simulink model "T2t"  (Simulink 8.4)
settings: Solver=ode45  StartTime=0.0  StopTime=10.0  RelTol=1e-3
undefined symbols (not defined in the file): T2t_facKThrValveReqCorr, T2t_facThrValveReqCorrEnable, T2t_facWastegateReqCorrEnable, T2t_KWastegateReqCorr, T2t_pManiReqMan, T2t_pManiReqMin, T2t_pManiReqOverride, T2t_pManiRes, T2t_ThrPosStart, T2t_ThrValve2WasteGateThreshold, T2t_ThrValveReqCorrMax, T2t_ThrValveReqCorrMin, T2t_tiTnThrValveReqCorr, T2t_tiTnWastegateReqCorr, T2t_tiTvThrValveReqCorr, T2t_tiTvWastegateReqCorr
libraries: simulink x5
settings Model: Creator=YAL9FE  LastModifiedBy=ric9fe
settings DebuggingCC: FcnCallInpInsideContextMsg=EnableAllAsWarning

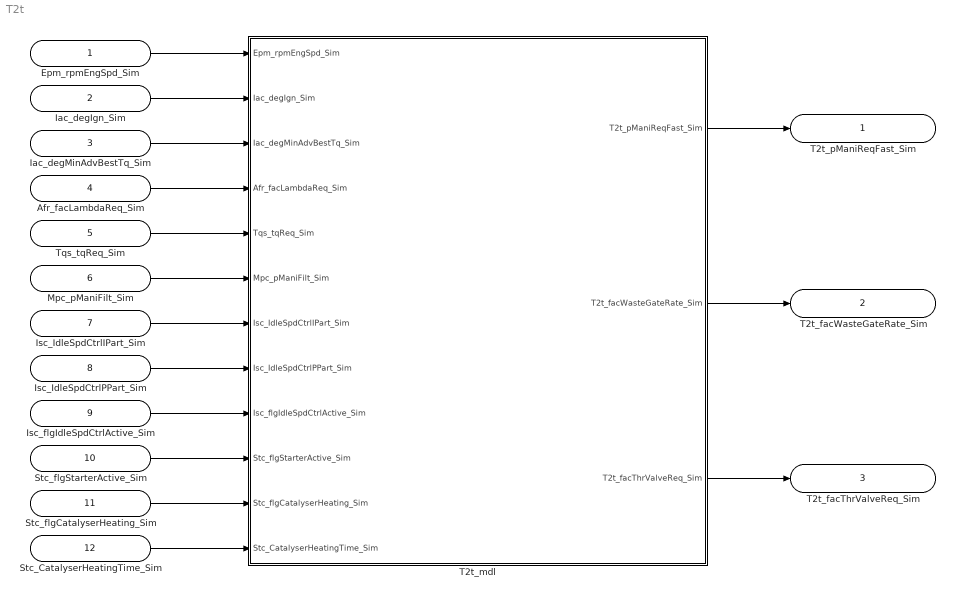
== system T2t ==
  Epm_rpmEngSpd_Sim : Inport
  Iac_degIgn_Sim : Inport  Port=2
  Iac_degMinAdvBestTq_Sim : Inport  Port=3
  Afr_facLambdaReq_Sim : Inport  Port=4
  Tqs_tqReq_Sim : Inport  Port=5
  Mpc_pManiFilt_Sim : Inport  Port=6
  Isc_IdleSpdCtrlIPart_Sim : Inport  Port=7
  Isc_IdleSpdCtrlPPart_Sim : Inport  Port=8
  Isc_flgIdleSpdCtrlActive_Sim : Inport  Port=9
  Stc_flgStarterActive_Sim : Inport  Port=10
  Stc_flgCatalyserHeating_Sim : Inport  Port=11
  Stc_CatalyserHeatingTime_Sim : Inport  Port=12
  T2t_mdl : Subsystem  mask(Functions){}
      mask help: Torque2Throttle
      mask Display:
      | image(imread('Torque2Throttle.jpg'))
      | port_label('input',1,'Epm_rpmEngSpd_Sim')
      | port_label('input',2,'Iac_degIgn_Sim')
      | port_label('input',3,'Iac_degMinAdvBestTq_Sim')
      | port_label('input',4,'Afr_facLambdaReq_Sim')
      | port_label('input',5,'Tqs_tqReq_Sim')
      | port_label('input',6,'Mpc_pManiFilt_Sim')
      | port_label('input',7,'Isc_IdleSpdCtrlIPart_Sim')
      | port_label('input',8,'Isc_IdleSpdCtrlPPart_Sim')
      | port_label('input',9,'Isc_flgIdleSpdCtrlActive_Sim')
      | port_label('input',10,'Stc_flgStarterActive_Sim')
      | port_label('input',11,'Stc_flgCatalyserHeating_Sim')
      | port_label('input',12,'Stc_CatalyserHeatingTime_Sim')
      | port_label('output',1,'T2t_pManiReqFast_Sim')
      | port_label('output',2,'T2t_facWasteGateRate_Sim')
      | port_label('output',3,'T2t_facThrValveReq_Sim')
  T2t_pManiReqFast_Sim : Outport
  T2t_facWasteGateRate_Sim : Outport  Port=2
  T2t_facThrValveReq_Sim : Outport  Port=3
  wires:
  Epm_rpmEngSpd_Sim/1 -> T2t_mdl/1(Epm_rpmEngSpd_Sim)
  Iac_degIgn_Sim/1 -> T2t_mdl/2(Iac_degIgn_Sim)
  Iac_degMinAdvBestTq_Sim/1 -> T2t_mdl/3(Iac_degMinAdvBestTq_Sim)
  Afr_facLambdaReq_Sim/1 -> T2t_mdl/4(Afr_facLambdaReq_Sim)
  Tqs_tqReq_Sim/1 -> T2t_mdl/5(Tqs_tqReq_Sim)
  Mpc_pManiFilt_Sim/1 -> T2t_mdl/6(Mpc_pManiFilt_Sim)
  Isc_IdleSpdCtrlIPart_Sim/1 -> T2t_mdl/7(Isc_IdleSpdCtrlIPart_Sim)
  Isc_IdleSpdCtrlPPart_Sim/1 -> T2t_mdl/8(Isc_IdleSpdCtrlPPart_Sim)
  Isc_flgIdleSpdCtrlActive_Sim/1 -> T2t_mdl/9(Isc_flgIdleSpdCtrlActive_Sim)
  Stc_flgStarterActive_Sim/1 -> T2t_mdl/10(Stc_flgStarterActive_Sim)
  Stc_flgCatalyserHeating_Sim/1 -> T2t_mdl/11(Stc_flgCatalyserHeating_Sim)
  Stc_CatalyserHeatingTime_Sim/1 -> T2t_mdl/12(Stc_CatalyserHeatingTime_Sim)
  T2t_mdl/1(T2t_pManiReqFast_Sim) -> T2t_pManiReqFast_Sim/1
  T2t_mdl/2(T2t_facWasteGateRate_Sim) -> T2t_facWasteGateRate_Sim/1
  T2t_mdl/3(T2t_facThrValveReq_Sim) -> T2t_facThrValveReq_Sim/1

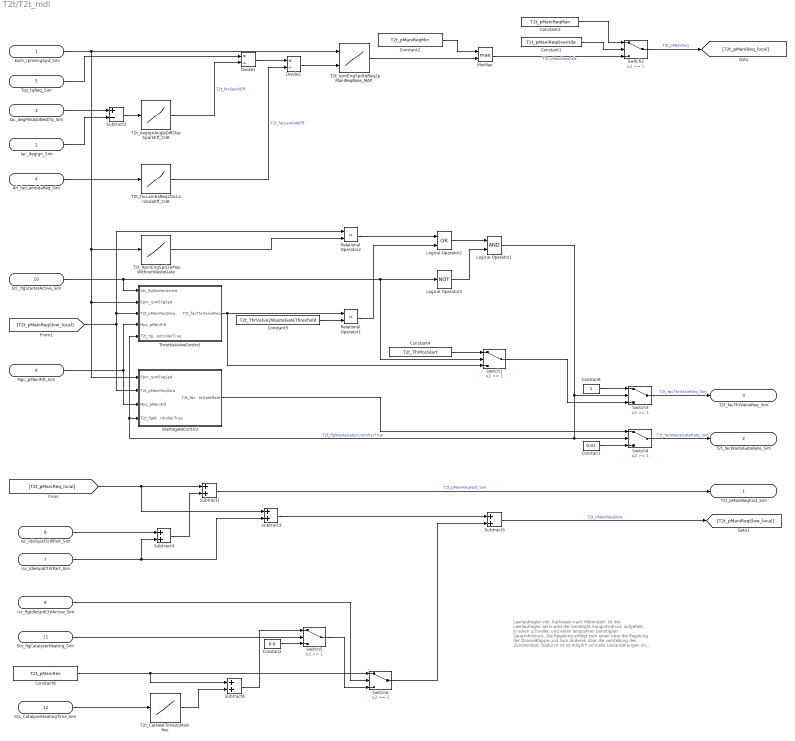
== system T2t/T2t_mdl ==
  note: Leerlaufregler inkl. Katheizen nach Motorstart:
      | Ist der Leerlaufregler aktiv wird der benötigte
      | Saugrohrdruck aufgeteilt, in einen schnellen
      | und einen langsamen benötigten Saugrohrdruck.
      | Die Regelung erfolgt zum einen über die
      | Regelung der Drosselklappe und zum anderen
      | über die verstellung des Zündwinkels.
      | Dadurch ist es möglich schnelle
      | Laständerungen im Leerlauf
      | durch Zündwinkeländerung auszuregeln.
      | Damit durch Zündwinkeländerung eine höhere
      | Momentenabgabe möglich ist, wird der
      | Saugrohrdruck erhöht um eine spätere
      | Zündung zu erhalten. Der
      | Zündwinkelwirkungsgrad wird niedriger.
      | Dadurch ist eine Momentenreserve vorhanden.
      |
      |
      | Der langsame Saugrohrdruck wird durch den
      | I-Anteil des Leerlaufreglers korrigiert.
      | Außerdem wird die Saugrohrdruckreserve addiert.
      | Der schnelle Saugrohrdruck wird durch den
      | P- und den I-Anteil des Leerlaufreglers korrigiert.
  Epm_rpmEngSpd_Sim : Inport
  Iac_degIgn_Sim : Inport  Port=2
  Iac_degMinAdvBestTq_Sim : Inport  Port=3
  Afr_facLambdaReq_Sim : Inport  Port=4
  Tqs_tqReq_Sim : Inport  Port=5
  Mpc_pManiFilt_Sim : Inport  Port=6
  Isc_IdleSpdCtrlIPart_Sim : Inport  Port=7
  Isc_IdleSpdCtrlPPart_Sim : Inport  Port=8
  Isc_flgIdleSpdCtrlActive_Sim : Inport  Port=9
  Stc_flgStarterActive_Sim : Inport  Port=10
  Stc_flgCatalyserHeating_Sim : Inport  Port=11
  Stc_CatalyserHeatingTime_Sim : Inport  Port=12
  Constan1 : Constant  Value=0.01  OutDataTypeStr=single
  Constan2 : Constant  Value=0.0  OutDataTypeStr=single
  Constan8 : Constant  OutDataTypeStr=single
  Constant1 : Constant  Value=T2t_pManiReqOverride
  Constant2 : Constant  Value=T2t_pManiReqMin
  Constant3 : Constant  Value=T2t_pManiReqMan
  Constant4 : Constant  Value=T2t_ThrPosStart
  Constant5 : Constant  Value=T2t_ThrValve2WasteGateThreshold
  Constant6 : Constant  Value=T2t_pManiRes
  Divide1 : Product  Inputs=*/  OutDataTypeStr=Inherit: Same as first input
  Divide2 : Product  Inputs=*/  OutDataTypeStr=Inherit: Same as first input
  Logical Operator1 : Logic  AllPortsSameDT=off  OutDataTypeStr=boolean
  Logical Operator2 : Logic  Operator=OR  AllPortsSameDT=off  OutDataTypeStr=boolean
  Logical Operator3 : Logic  Operator=NOT  AllPortsSameDT=off  OutDataTypeStr=boolean
  MinMax : MinMax  Function=max  Inputs=2
  Relational Operator1 : RelationalOperator  Operator=>  OutDataTypeStr=boolean
  Relational Operator2 : RelationalOperator  Operator=>  OutDataTypeStr=boolean
  Subtract{1,3..6} (5 alike) : Sum  OutDataTypeStr=Inherit: Same as first input
  Subtract2 : Sum  Inputs=+-  OutDataTypeStr=Inherit: Same as first input
  Switch{1..6} (6 alike) : Switch  Threshold=1
  T2t_CatHeatTime2pManiRes : Lookup_n-D  NumberOfTableDimensions=1  BreakpointsForDimension1=[1:3]  Table=[2 6 9]  ExtrapMethod=Clip  InputSameDT=on
  T2t_RpmEngSpd2pMaxWithoutWasteGate : Lookup_n-D  NumberOfTableDimensions=1  BreakpointsForDimension1=[1:3]  Table=[6 4 3]  ExtrapMethod=Clip  InputSameDT=on
  T2t_degIgnAngleDiff2facSparkEff_CUR : Lookup_n-D  NumberOfTableDimensions=1  BreakpointsForDimension1=[1:3]  Table=[6 3 9]  ExtrapMethod=Clip  InputSameDT=on
  T2t_facLambaReq2facLambdaEff_CUR : Lookup_n-D  NumberOfTableDimensions=1  BreakpointsForDimension1=[1:3]  Table=[4 7 8]  ExtrapMethod=Clip  InputSameDT=on
  T2t_rpmEngSpdtqReq2pManiReqBase_MAP : Lookup_n-D  BreakpointsForDimension1=[1:3]  BreakpointsForDimension2=[1:3]  ExtrapMethod=Clip  InputSameDT=on
  ThrottleValveControl : Subsystem
  WastegateControl : Subsystem
  T2t_pManiReqFast_Sim : Outport
  T2t_facWasteGateRate_Sim : Outport  Port=2
  T2t_facThrValveReq_Sim : Outport  Port=3
  wires:
  Constant1/1 -> Switch2/2
  Constant3/1 -> Switch2/1
  MinMax/1 -> Switch2/3  "T2t_pManiReqCalc"
  Constant2/1 -> MinMax/1
  T2t_rpmEngSpdtqReq2pManiReqBase_MAP/1 -> MinMax/2
  Switch2/1 -> [T2t_pManiReq_local]  "T2t_pManiReq"
  Divide2/1 -> T2t_rpmEngSpdtqReq2pManiReqBase_MAP/2
  Divide1/1 -> Divide2/1
  Epm_rpmEngSpd_Sim/1 -> T2t_rpmEngSpdtqReq2pManiReqBase_MAP/1, T2t_RpmEngSpd2pMaxWithoutWasteGate/1, ThrottleValveControl/2(Epm_rpmEngSpd), WastegateControl/1(Epm_rpmEngSpd)
  Tqs_tqReq_Sim/1 -> Divide1/1
  Iac_degMinAdvBestTq_Sim/1 -> Subtract2/1
  Iac_degIgn_Sim/1 -> Subtract2/2
  Subtract2/1 -> T2t_degIgnAngleDiff2facSparkEff_CUR/1
  T2t_degIgnAngleDiff2facSparkEff_CUR/1 -> Divide1/2  "T2t_facSparkEff"
  Afr_facLambdaReq_Sim/1 -> T2t_facLambaReq2facLambdaEff_CUR/1
  T2t_facLambaReq2facLambdaEff_CUR/1 -> Divide2/2  "T2t_facLambdaEff"
  T2t_RpmEngSpd2pMaxWithoutWasteGate/1 -> Relational Operator2/2
  Relational Operator2/1 -> Logical Operator2/1
  Stc_flgStarterActive_Sim/1 -> ThrottleValveControl/1(Stc_flgStarterActive), Switch1/2, Logical Operator3/1
  Logical Operator2/1 -> Logical Operator1/1
  Logical Operator3/1 -> Logical Operator1/2
  Constant4/1 -> Switch1/1
  Logical Operator1/1 -> Switch3/2, Switch4/2, ThrottleValveControl/5(T2t_flgWasteGateControllerTrue), WastegateControl/4(T2t_flgWasteGateControllerTrue)  "T2t_flgWasteGateControllerTrue"
  Constan8/1 -> Switch3/1
  Switch1/1 -> Switch3/3
  Switch3/1 -> T2t_facThrValveReq_Sim/1  "T2t_facThrValveReq_Sim"
  Relational Operator1/1 -> Logical Operator2/2
  Constant5/1 -> Relational Operator1/2
  Switch4/1 -> T2t_facWasteGateRate_Sim/1  "T2t_facWasteGateRate_Sim"
  Constan1/1 -> Switch4/3
  [T2t_pManiReq_local] -> Subtract1/1, Subtract3/1
  Subtract4/1 -> Subtract1/2
  Isc_IdleSpdCtrlPPart_Sim/1 -> Subtract4/1
  Isc_IdleSpdCtrlIPart_Sim/1 -> Subtract4/2, Subtract3/2
  Subtract1/1 -> T2t_pManiReqFast_Sim/1  "T2t_pManiReqFast_Sim"
  [T2t_pManiReqSlow_local] -> Relational Operator2/1, ThrottleValveControl/3(T2t_pManiReqSlow), WastegateControl/2(T2t_pManiReqSlow)
  Subtract3/1 -> Subtract5/1
  Subtract5/1 -> [T2t_pManiReqSlow_local]  "T2t_pManiReqSlow"
  Stc_CatalyserHeatingTime_Sim/1 -> T2t_CatHeatTime2pManiRes/1
  Constant6/1 -> Subtract6/1, Switch6/1
  T2t_CatHeatTime2pManiRes/1 -> Subtract6/2
  Constan2/1 -> Switch5/3
  Stc_flgCatalyserHeating_Sim/1 -> Switch5/2
  Subtract6/1 -> Switch5/1
  Switch5/1 -> Switch6/3
  Isc_flgIdleSpdCtrlActive_Sim/1 -> Switch6/2
  Switch6/1 -> Subtract5/2
  ThrottleValveControl/1(T2t_facThrValveReq) -> Relational Operator1/1, Switch1/3
  Mpc_pManiFilt_Sim/1 -> ThrottleValveControl/4(Mpc_pManiFilt), WastegateControl/3(Mpc_pManiFilt)
  WastegateControl/1(T2t_facWasteGateRate) -> Switch4/1

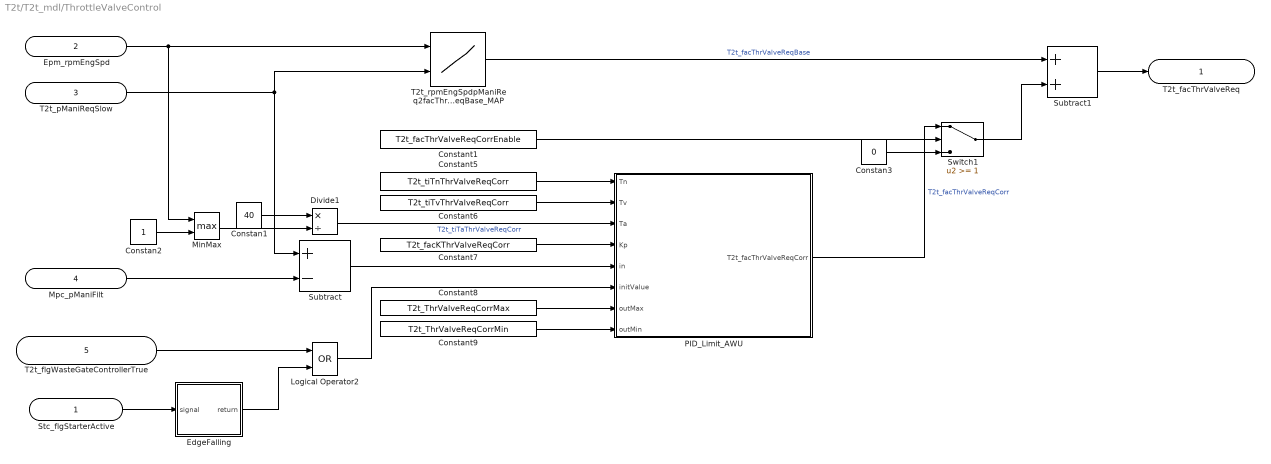
== system T2t/T2t_mdl/ThrottleValveControl ==
  Stc_flgStarterActive : Inport
  Epm_rpmEngSpd : Inport  Port=2
  T2t_pManiReqSlow : Inport  Port=3
  Mpc_pManiFilt : Inport  Port=4
  T2t_flgWasteGateControllerTrue : Inport  Port=5
  Constan1 : Constant  Value=40  OutDataTypeStr=single
  Constan2 : Constant  OutDataTypeStr=single
  Constan3 : Constant  Value=0  OutDataTypeStr=single
  Constant1 : Constant  Value=T2t_facThrValveReqCorrEnable
  Constant5 : Constant  Value=T2t_tiTnThrValveReqCorr
  Constant6 : Constant  Value=T2t_tiTvThrValveReqCorr
  Constant7 : Constant  Value=T2t_facKThrValveReqCorr
  Constant8 : Constant  Value=T2t_ThrValveReqCorrMax
  Constant9 : Constant  Value=T2t_ThrValveReqCorrMin
  Divide1 : Product  Inputs=*/  OutDataTypeStr=Inherit: Same as first input
  EdgeFalling : Subsystem
      mask help: EdgeFalling
      mask Display: image(imread('EdgeFalling.jpg'))
  Logical Operator2 : Logic  Operator=OR  AllPortsSameDT=off  OutDataTypeStr=boolean
  MinMax : MinMax  Function=max  Inputs=2
  PID_Limit_AWU : Subsystem
      mask help: PID_Limit_AWU
      mask Display: image(imread('PID_Limit_AWU.jpg'))
  Subtract : Sum  Inputs=+-  OutDataTypeStr=Inherit: Same as first input
  Subtract1 : Sum  OutDataTypeStr=Inherit: Same as first input
  Switch1 : Switch  Threshold=1
  T2t_rpmEngSpdpManiReq2facThrValveReqBase_MAP : Lookup_n-D  BreakpointsForDimension1=[1:3]  BreakpointsForDimension2=[1:3]  ExtrapMethod=Clip  InputSameDT=on
  T2t_facThrValveReq : Outport
  wires:
  Constant5/1 -> PID_Limit_AWU/1(Tn)
  Subtract/1 -> PID_Limit_AWU/5(in)
  Constant6/1 -> PID_Limit_AWU/2(Tv)
  Constant7/1 -> PID_Limit_AWU/4(Kp)
  Constant8/1 -> PID_Limit_AWU/7(outMax)
  Constant9/1 -> PID_Limit_AWU/8(outMin)
  Epm_rpmEngSpd/1 -> T2t_rpmEngSpdpManiReq2facThrValveReqBase_MAP/1, MinMax/1
  T2t_pManiReqSlow/1 -> T2t_rpmEngSpdpManiReq2facThrValveReqBase_MAP/2, Subtract/1
  T2t_rpmEngSpdpManiReq2facThrValveReqBase_MAP/1 -> Subtract1/1  "T2t_facThrValveReqBase"
  Subtract1/1 -> T2t_facThrValveReq/1
  Constant1/1 -> Switch1/2
  Switch1/1 -> Subtract1/2
  Mpc_pManiFilt/1 -> Subtract/2
  T2t_flgWasteGateControllerTrue/1 -> Logical Operator2/1
  Stc_flgStarterActive/1 -> EdgeFalling/1(signal)
  EdgeFalling/1(return) -> Logical Operator2/2
  Logical Operator2/1 -> PID_Limit_AWU/6(initValue)
  Divide1/1 -> PID_Limit_AWU/3(Ta)  "T2t_tiTaThrValveReqCorr"
  Constan1/1 -> Divide1/1
  MinMax/1 -> Divide1/2
  Constan2/1 -> MinMax/2
  Constan3/1 -> Switch1/3
  PID_Limit_AWU/1(T2t_facThrValveReqCorr) -> Switch1/1  "T2t_facThrValveReqCorr"

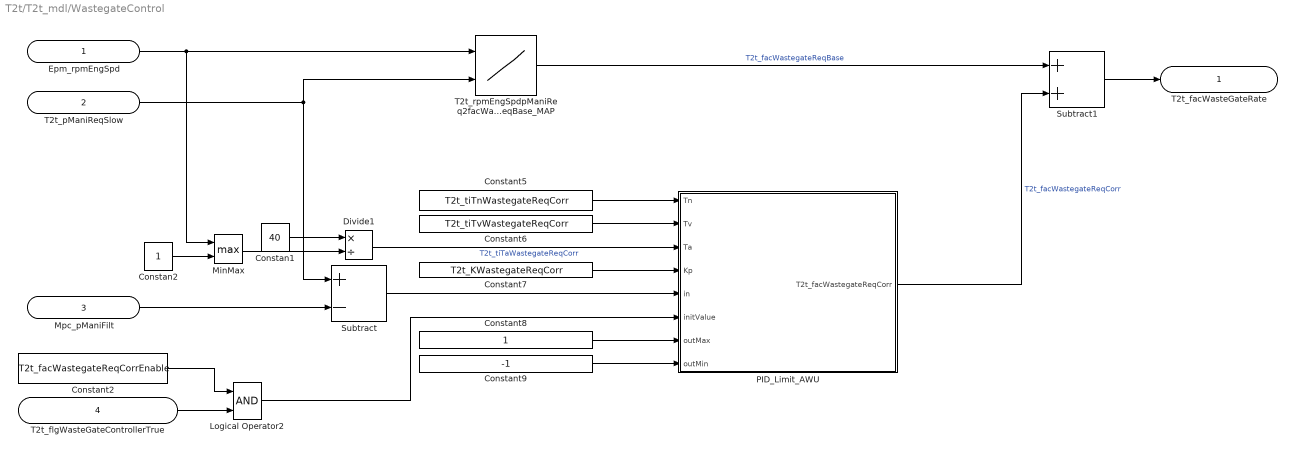
== system T2t/T2t_mdl/WastegateControl ==
  Epm_rpmEngSpd : Inport
  T2t_pManiReqSlow : Inport  Port=2
  Mpc_pManiFilt : Inport  Port=3
  T2t_flgWasteGateControllerTrue : Inport  Port=4
  Constan1 : Constant  Value=40  OutDataTypeStr=single
  Constan2 : Constant  OutDataTypeStr=single
  Constant2 : Constant  Value=T2t_facWastegateReqCorrEnable
  Constant5 : Constant  Value=T2t_tiTnWastegateReqCorr
  Constant6 : Constant  Value=T2t_tiTvWastegateReqCorr
  Constant7 : Constant  Value=T2t_KWastegateReqCorr
  Constant8 : Constant
  Constant9 : Constant  Value=-1
  Divide1 : Product  Inputs=*/  OutDataTypeStr=Inherit: Same as first input
  Logical Operator2 : Logic  AllPortsSameDT=off  OutDataTypeStr=boolean
  MinMax : MinMax  Function=max  Inputs=2
  PID_Limit_AWU : Subsystem
      mask help: PID_Limit_AWU
      mask Display: image(imread('PID_Limit_AWU.jpg'))
  Subtract : Sum  Inputs=+-  OutDataTypeStr=Inherit: Same as first input
  Subtract1 : Sum  OutDataTypeStr=Inherit: Same as first input
  T2t_rpmEngSpdpManiReq2facWastegateReqBase_MAP : Lookup_n-D  BreakpointsForDimension1=[1:3]  BreakpointsForDimension2=[1:3]  ExtrapMethod=Clip  InputSameDT=on
  T2t_facWasteGateRate : Outport
  wires:
  Constan2/1 -> MinMax/2
  MinMax/1 -> Divide1/2
  Constan1/1 -> Divide1/1
  Divide1/1 -> PID_Limit_AWU/3(Ta)  "T2t_tiTaWastegateReqCorr"
  Logical Operator2/1 -> PID_Limit_AWU/6(initValue)
  Mpc_pManiFilt/1 -> Subtract/2
  Subtract1/1 -> T2t_facWasteGateRate/1
  T2t_rpmEngSpdpManiReq2facWastegateReqBase_MAP/1 -> Subtract1/1  "T2t_facWastegateReqBase"
  T2t_pManiReqSlow/1 -> Subtract/1, T2t_rpmEngSpdpManiReq2facWastegateReqBase_MAP/2
  Epm_rpmEngSpd/1 -> MinMax/1, T2t_rpmEngSpdpManiReq2facWastegateReqBase_MAP/1
  Constant9/1 -> PID_Limit_AWU/8(outMin)
  Constant8/1 -> PID_Limit_AWU/7(outMax)
  Constant7/1 -> PID_Limit_AWU/4(Kp)
  Constant6/1 -> PID_Limit_AWU/2(Tv)
  Subtract/1 -> PID_Limit_AWU/5(in)
  Constant5/1 -> PID_Limit_AWU/1(Tn)
  T2t_flgWasteGateControllerTrue/1 -> Logical Operator2/2
  Constant2/1 -> Logical Operator2/1
  PID_Limit_AWU/1(T2t_facWastegateReqCorr) -> Subtract1/2  "T2t_facWastegateReqCorr"

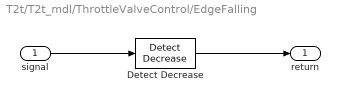
== system T2t/T2t_mdl/ThrottleValveControl/EdgeFalling ==
  signal : Inport
  Detect Decrease : simulink/Logic and Bit Operations/Detect Decrease  vinit=0.0  InputProcessing=Inherited  OutDataTypeStr=boolean
  return : Outport
  wires:
  Detect Decrease/1 -> return/1
  signal/1 -> Detect Decrease/1

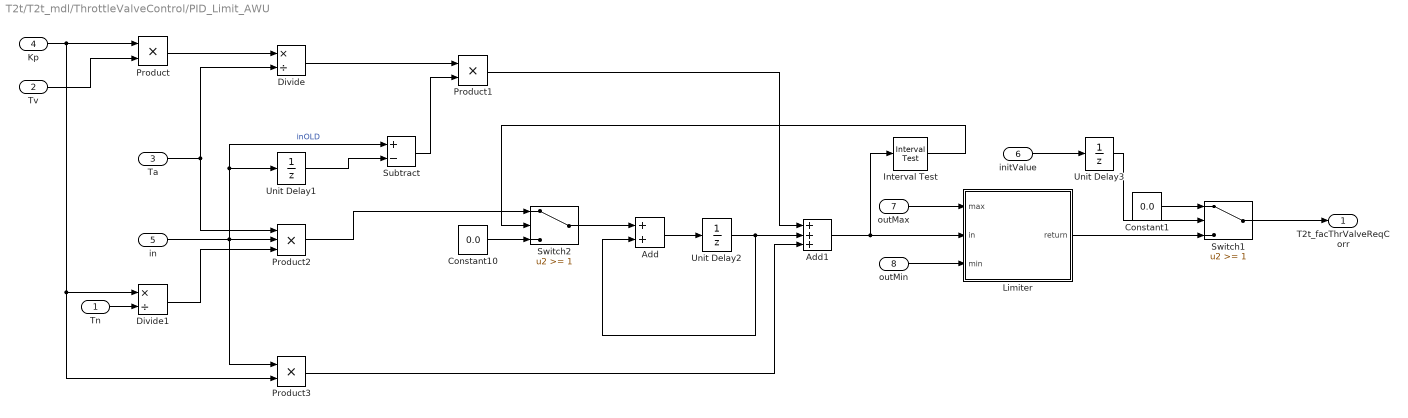
== system T2t/T2t_mdl/ThrottleValveControl/PID_Limit_AWU ==
  Tn : Inport
  Tv : Inport  Port=2
  Ta : Inport  Port=3
  Kp : Inport  Port=4
  in : Inport  Port=5
  initValue : Inport  Port=6
  outMax : Inport  Port=7
  outMin : Inport  Port=8
  Add : Sum  OutDataTypeStr=Inherit: Same as first input
  Add1 : Sum  Inputs=+++  OutDataTypeStr=Inherit: Same as first input
  Constant1 : Constant  Value=0.0  OutDataTypeStr=single
  Constant10 : Constant  Value=0.0  OutDataTypeStr=single
  Divide : Product  Inputs=*/  OutDataTypeStr=Inherit: Same as first input
  Divide1 : Product  Inputs=*/  OutDataTypeStr=Inherit: Same as first input
  Interval Test : simulink/Logic and Bit Operations/Interval Test  IntervalClosedRight=on  uplimit=T2t_ThrValveReqCorrMax  IntervalClosedLeft=on  lowlimit=T2t_ThrValveReqCorrMin  OutDataTypeStr=boolean
  Limiter : Subsystem
      mask help: Limiter
      mask Display: image(imread('Limiter.jpg'))
  Product : Product  OutDataTypeStr=Inherit: Same as first input
  Product1 : Product  OutDataTypeStr=Inherit: Same as first input
  Product2 : Product  Inputs=3  OutDataTypeStr=Inherit: Same as first input
  Product3 : Product  OutDataTypeStr=Inherit: Same as first input
  Subtract : Sum  Inputs=+-  OutDataTypeStr=Inherit: Same as first input
  Switch1 : Switch  Threshold=1
  Switch2 : Switch  Threshold=1
  Unit Delay1 : UnitDelay  SampleTime=-1
  Unit Delay2 : UnitDelay  SampleTime=-1
  Unit Delay3 : UnitDelay  SampleTime=-1
  T2t_facThrValveReqCorr : Outport
  wires:
  Constant10/1 -> Switch2/3
  Product2/1 -> Switch2/1
  Interval Test/1 -> Switch2/2
  Unit Delay2/1 -> Add/2, Add1/2
  Add/1 -> Unit Delay2/1
  Unit Delay1/1 -> Subtract/2
  Kp/1 -> Product/1, Product3/2, Divide1/1
  Tv/1 -> Product/2
  Product/1 -> Divide/1
  Ta/1 -> Product2/1, Divide/2
  Divide/1 -> Product1/1
  Tn/1 -> Divide1/2
  in/1 -> Product2/2, Product3/1, Subtract/1, Unit Delay1/1  "inOLD"
  Divide1/1 -> Product2/3
  Subtract/1 -> Product1/2
  Switch2/1 -> Add/1
  Product3/1 -> Add1/3
  Product1/1 -> Add1/1
  Add1/1 -> Limiter/2(in), Interval Test/1
  outMin/1 -> Limiter/3(min)
  outMax/1 -> Limiter/1(max)
  Switch1/1 -> T2t_facThrValveReqCorr/1
  Constant1/1 -> Switch1/1
  Limiter/1(return) -> Switch1/3
  initValue/1 -> Unit Delay3/1
  Unit Delay3/1 -> Switch1/2

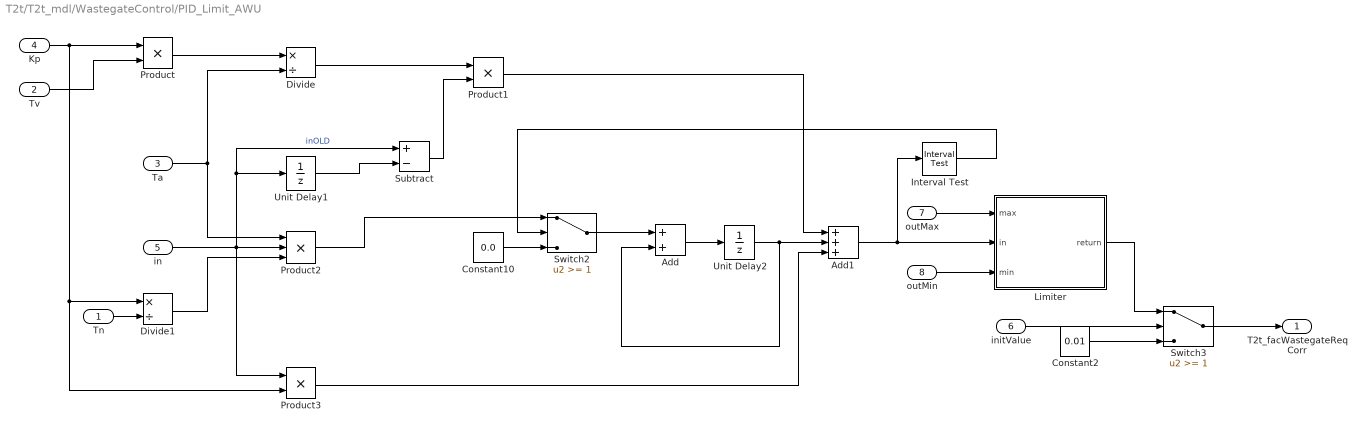
== system T2t/T2t_mdl/WastegateControl/PID_Limit_AWU ==
  Tn : Inport
  Tv : Inport  Port=2
  Ta : Inport  Port=3
  Kp : Inport  Port=4
  in : Inport  Port=5
  initValue : Inport  Port=6
  outMax : Inport  Port=7
  outMin : Inport  Port=8
  Add : Sum  OutDataTypeStr=Inherit: Same as first input
  Add1 : Sum  Inputs=+++  OutDataTypeStr=Inherit: Same as first input
  Constant10 : Constant  Value=0.0  OutDataTypeStr=single
  Constant2 : Constant  Value=0.01  OutDataTypeStr=single
  Divide : Product  Inputs=*/  OutDataTypeStr=Inherit: Same as first input
  Divide1 : Product  Inputs=*/  OutDataTypeStr=Inherit: Same as first input
  Interval Test : simulink/Logic and Bit Operations/Interval Test  IntervalClosedRight=on  uplimit=1  IntervalClosedLeft=on  lowlimit=-1  OutDataTypeStr=boolean
  Limiter : Subsystem
      mask help: Limiter
      mask Display: image(imread('Limiter.jpg'))
  Product : Product  OutDataTypeStr=Inherit: Same as first input
  Product1 : Product  OutDataTypeStr=Inherit: Same as first input
  Product2 : Product  Inputs=3  OutDataTypeStr=Inherit: Same as first input
  Product3 : Product  OutDataTypeStr=Inherit: Same as first input
  Subtract : Sum  Inputs=+-  OutDataTypeStr=Inherit: Same as first input
  Switch2 : Switch  Threshold=1
  Switch3 : Switch  Threshold=1
  Unit Delay1 : UnitDelay  SampleTime=-1
  Unit Delay2 : UnitDelay  SampleTime=-1
  T2t_facWastegateReqCorr : Outport
  wires:
  outMax/1 -> Limiter/1(max)
  outMin/1 -> Limiter/3(min)
  Add1/1 -> Interval Test/1, Limiter/2(in)
  Product1/1 -> Add1/1
  Product3/1 -> Add1/3
  Switch2/1 -> Add/1
  Subtract/1 -> Product1/2
  Divide1/1 -> Product2/3
  in/1 -> Unit Delay1/1, Subtract/1, Product3/1, Product2/2  "inOLD"
  Tn/1 -> Divide1/2
  Divide/1 -> Product1/1
  Ta/1 -> Divide/2, Product2/1
  Product/1 -> Divide/1
  Tv/1 -> Product/2
  Kp/1 -> Divide1/1, Product3/2, Product/1
  Unit Delay1/1 -> Subtract/2
  Add/1 -> Unit Delay2/1
  Unit Delay2/1 -> Add1/2, Add/2
  Interval Test/1 -> Switch2/2
  Product2/1 -> Switch2/1
  Constant10/1 -> Switch2/3
  Constant2/1 -> Switch3/3
  initValue/1 -> Switch3/2
  Switch3/1 -> T2t_facWastegateReqCorr/1
  Limiter/1(return) -> Switch3/1

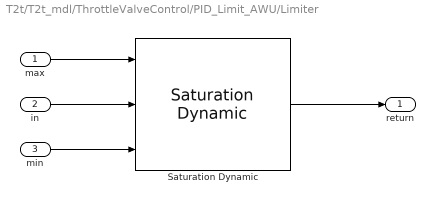
== system T2t/T2t_mdl/ThrottleValveControl/PID_Limit_AWU/Limiter ==
  max : Inport
  in : Inport  Port=2
  min : Inport  Port=3
  Saturation Dynamic : simulink/Discontinuities/Saturation Dynamic  OutMin=[]  OutMax=[]  OutDataTypeStr=Inherit: Same as second input  OutDataType=fixdt(1, 16)  OutScaling=2^-10  DoSatur=off
  return : Outport
  wires:
  max/1 -> Saturation Dynamic/1
  in/1 -> Saturation Dynamic/2
  min/1 -> Saturation Dynamic/3
  Saturation Dynamic/1 -> return/1

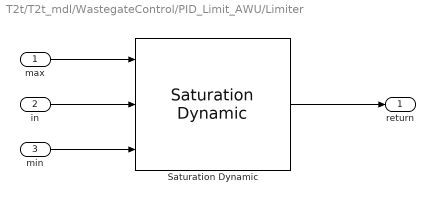
== system T2t/T2t_mdl/WastegateControl/PID_Limit_AWU/Limiter ==
  max : Inport
  in : Inport  Port=2
  min : Inport  Port=3
  Saturation Dynamic : simulink/Discontinuities/Saturation Dynamic  OutMin=[]  OutMax=[]  OutDataTypeStr=Inherit: Same as second input  OutDataType=fixdt(1, 16)  OutScaling=2^-10  DoSatur=off
  return : Outport
  wires:
  Saturation Dynamic/1 -> return/1
  min/1 -> Saturation Dynamic/3
  in/1 -> Saturation Dynamic/2
  max/1 -> Saturation Dynamic/1
